simulink model "SIMULINK_MasaTlumikSprezyna_toWorkspace"  (R2024b)
settings: Solver=FixedStepAuto  StartTime=0.0  StopTime=10.0  FixedStep=0.001  RelTol=1e-3
settings Model: Creator=pawel  LastModifiedBy=pawel

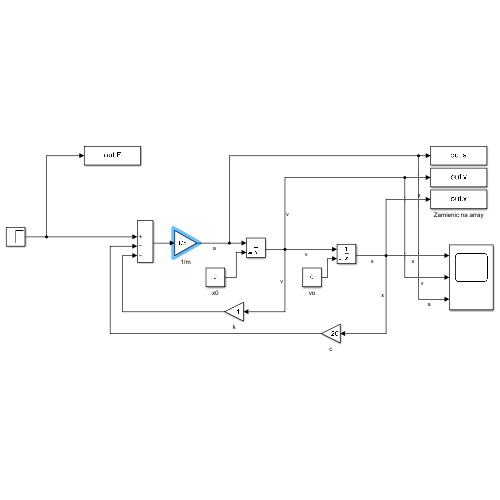
[thumbnail: Simulink's stored preview of the top-level diagram]
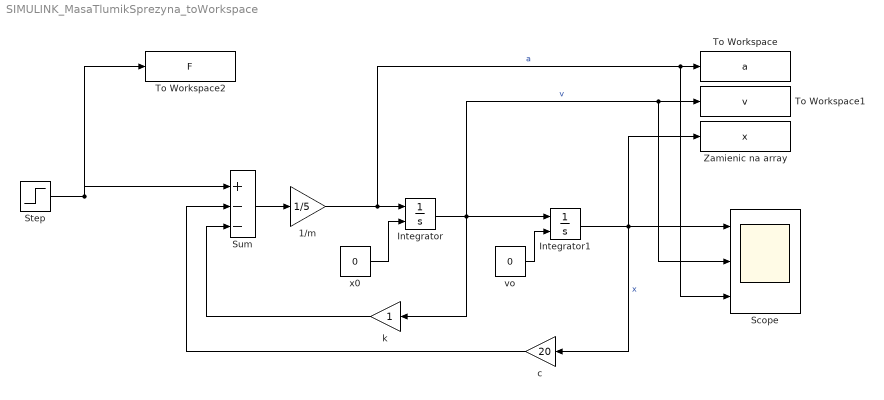
== system SIMULINK_MasaTlumikSprezyna_toWorkspace ==
  1/m : Gain  Gain=1/5
  Integrator : Integrator  InitialConditionSource=external  InitialCondition=1
  Integrator1 : Integrator  InitialConditionSource=external  InitialCondition=10
  Scope : Scope  NumInputPorts=3
  Step : Step  SampleTime=0
  Sum : Sum  Inputs=|+--
  To Workspace : ToWorkspace  VariableName=a  SampleTime=-1
  To Workspace1 : ToWorkspace  VariableName=v  SampleTime=-1
  To Workspace2 : ToWorkspace  VariableName=F  SampleTime=-1
  Zamienic na array : ToWorkspace  VariableName=x  SampleTime=-1
  c : Gain  Gain=20
  k : Gain
  vo : Constant  Value=0
  x0 : Constant  Value=0
  wires:
  Step/1 -> To Workspace2/1, Sum/1
  Sum/1 -> 1/m/1
  Integrator/1 -> Scope/2, To Workspace1/1, Integrator1/1, k/1  "v"
  Integrator1/1 -> Zamienic na array/1, Scope/1, c/1  "x"
  c/1 -> Sum/2
  k/1 -> Sum/3
  x0/1 -> Integrator/2
  vo/1 -> Integrator1/2
  1/m/1 -> Scope/3, To Workspace/1, Integrator/1  "a"
